simulink model "c1_soft_border"  (R2021b)
settings: Solver=FixedStepDiscrete  StartTime=0.0  StopTime=Inf  FixedStep=sampleTime  RelTol=1e-3  EnableMultiTasking=on
InitFcn:
  | sampleTime = 0.05;
  | nMedianSize=3;
  | % Robot parameters
  | wheelRadius = 0.025;
  | robotRadius = 0.15;
  | 
  | % Lidar parameters
  | sensorOffset = [0,0];
  | scanAngles = linspace(-pi/2,pi/2,9)';
  | maxRange = 5;
  | 
  | %%%%%%
  | ks=-1;
  | 
  | %初始位置
  | x_1_0=0;
  | y_1_0=0;
  | yaw_1_0=0;
  | 
  | x_2_0=0;
  | y_2_0=0.3;
  | yaw_2_0=0;
  | 
  | x_3_0=0;
  | y_3_0=0.6;
  | yaw_3_0=0;
  | 
  | x_4_0=0;
  | y_4_0=0.9;
  | yaw_4_0=0;
  | 
  | 
  | A=0.3;
  | C=1.7;
  | B=(A+C)/2;
  | 
  | wp1=[A,A; B,A;  C,A; C,B;C,C; B,C; A,C;A,B];
  | t=0:0.5:5;
  | Ax=0.8;Ay=0.8;f=2*pi/10;
  | Xd=Ax*sin(2*f*t)+1;
  | Yd=Ay*sin(f*t)+1;
  | WAY_P1=[Xd',Yd'];
  | Ax=0.8;Ay=0.8;f=2*pi/10;
  | Xd=Ax*sin(2*f*t)+1;
  | Yd=-Ay*sin(f*t)+1;
  | WAY_P2=[Xd',Yd'];
  | WAY_P=[WAY_P1(1:end-1,:);WAY_P2(1:end-1,:)];
  | WAY_P=[WAY_P(1:15,:);1,0.5;WAY_P(17:end,:)];
undefined symbols (not defined in the file): Angular, DiscIntNeverNeededParam, Linear
libraries: robotlib x4, dspstat3 x3
settings Model: Creator=The MathWorks, Inc.  LastModifiedBy=FCS
settings SolverCC: AlgebraicLoopSolver=TrustRegion
settings DataIOCC: LimitDataPoints=on  SaveFormat=Array  ReturnWorkspaceOutputs=off
settings OptimizationCC: EnhancedBackFolding=on  PassReuseOutputArgsAs=Individual arguments  ZeroExternalMemoryAtStartup=off  ZeroInternalMemoryAtStartup=off  MaxStackSize=64  OptimizeBlockOrder=speed  DifferentSizesBufferReuse=on  OptimizationCustomize=off  EfficientTunableParamExpr=on
settings DebuggingCC: SolverPrmCheckMsg=warning  ParameterTunabilityLossMsg=error  SFUnexpectedBacktrackingDiag=warning  SFNoUnconditionalDefaultTransitionDiag=warning  SFExecutionAtInitializationDiag=none  SFMachineParentedDataDiag=warning  ArithmeticOperatorsInVariantConditions=warning
settings HardwareCC: ProdBitPerPointer=32  ProdBitPerSizeT=32  ProdBitPerPtrDiffT=32  ProdLargestAtomicFloat=None  ProdIntDivRoundTo=Undefined  ProdEndianess=Unspecified  ProdWordSize=32  ProdHWDeviceType=Generic->Unspecified (assume 32-bit Generic)  TargetHWDeviceType=Generic->Unspecified (assume 32-bit Generic)
settings ModelReferenceCC: PropagateSignalLabelsOutOfModel=off
settings SFSimCC: SimUseLocalCustomCode=off  MATLABDynamicMemAlloc=off  CustomCodeUndefinedFunction=UseInterfaceOnly  SimTargetLang=C++
settings RTWCC: Description=Embedded Coder  SystemTargetFile=ert.tlc  HardwareBoard=Robot Operating System (ROS)  TLCOptions="-aInlineSetEventsForThisBaseRateFcn=TLC_FALSE -aSuppressMultiTaskScheduler=TLC_FALSE  -aRateBasedStepFcn=0"  TemplateMakefile=ert_default_tmf  RTWUseLocalCustomCode=off  Toolchain=Catkin  TargetLang=C++
settings CodeAppCC: ForceParamTrailComments=on  IgnoreCustomStorageClasses=off  OperatorAnnotations=on  SimulinkDataObjDesc=on  SFDataObjDesc=on  InsertBlockDesc=on
settings ERTTargetCC: SupportVariableSizeSignals=on
settings ConfigComp: CovMetricSettings=dw  CovSaveCumulativeToWorkspaceVar=on  CovSaveSingleToWorkspaceVar=on  CovExternalEMLEnable=off  CovSFcnEnable=off

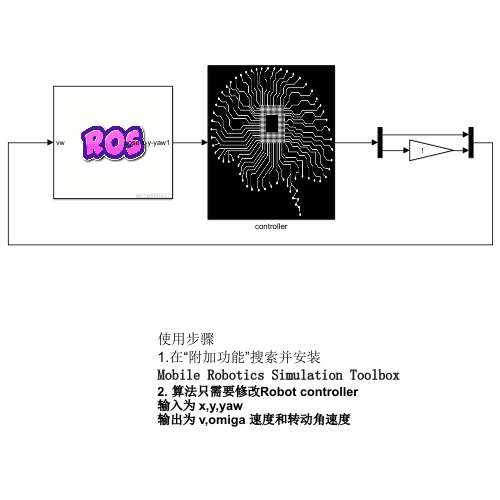
[thumbnail: Simulink's stored preview of the top-level diagram]
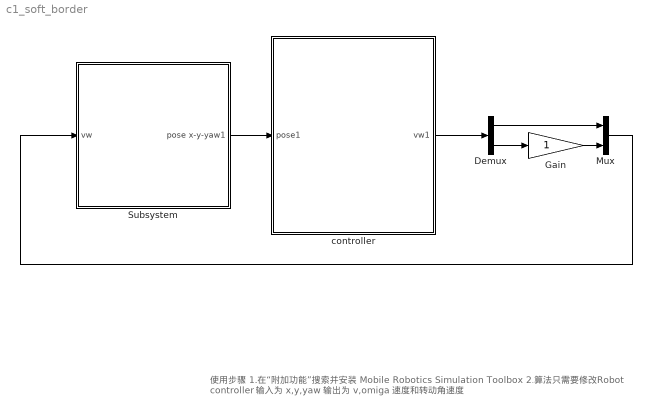
== system c1_soft_border ==
  note: 使用步骤
      | 1.在“附加功能”搜索并安装
      | Mobile Robotics Simulation Toolbox
      | 2. 算法只需要修改Robot controller
      | 输入为 x,y,yaw
      | 输出为 v,omiga 速度和转动角速度
  Demux : Demux  Outputs=2
  Gain : Gain
  Mux : Mux  Inputs=2
  Subsystem : Subsystem
      mask Display: image('$imagefile'); % 使用工具条上的 "编辑图像" 进行更改。
  controller : Subsystem
      mask Display: image('$imagefile'); % 使用工具条上的 "编辑图像" 进行更改。
  wires:
  Mux/1 -> Subsystem/1(vw)
  Gain/1 -> Mux/2
  Subsystem/1(pose x-y-yaw1) -> controller/1(pose1)
  Demux/2 -> Gain/1
  Demux/1 -> Mux/1
  controller/1(vw1) -> Demux/1

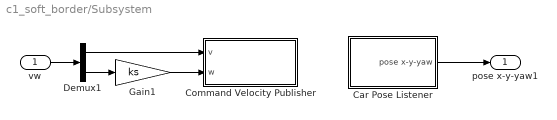
== system c1_soft_border/Subsystem ==
  vw : Inport
  Car Pose Listener : Subsystem
  Command Velocity Publisher : Subsystem
  Demux1 : Demux  Outputs=2
  Gain1 : Gain  Gain=ks
  pose x-y-yaw1 : Outport
  wires:
  vw/1 -> Demux1/1
  Gain1/1 -> Command Velocity Publisher/2(w)
  Demux1/2 -> Gain1/1
  Demux1/1 -> Command Velocity Publisher/1(v)
  Car Pose Listener/1(pose x-y-yaw) -> pose x-y-yaw1/1

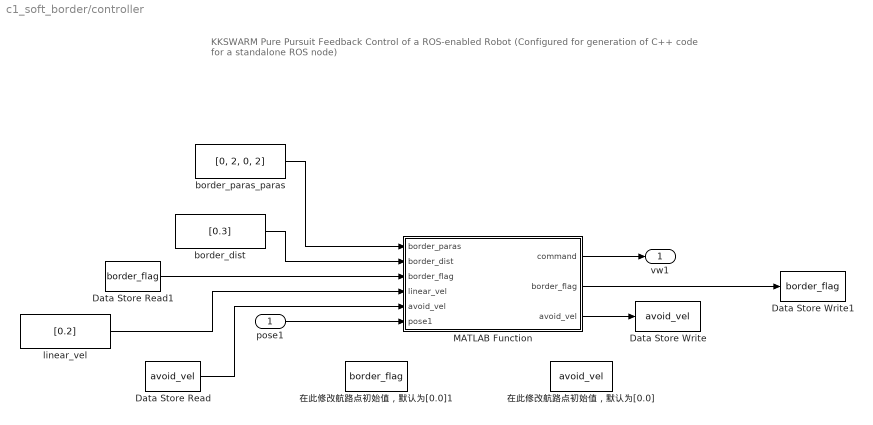
== system c1_soft_border/controller ==
  note: KKSWARM Pure Pursuit Feedback Control of a ROS-enabled Robot
      | (Configured for generation of C++ code for a standalone ROS node)
  pose1 : Inport
  Data Store Read : DataStoreRead  DataStoreName=avoid_vel  IndexOptions=Index vector (dialog)  Indices=1  OutputSizes=1
  Data Store Read1 : DataStoreRead  DataStoreName=border_flag  IndexOptions=Index vector (dialog)  Indices=1  OutputSizes=1
  Data Store Write : DataStoreWrite  DataStoreName=avoid_vel  IndexOptions=Index vector (dialog)  Indices=1  OutputSizes=1
  Data Store Write1 : DataStoreWrite  DataStoreName=border_flag  IndexOptions=Index vector (dialog)  Indices=1  OutputSizes=1
  MATLAB Function : MATLAB Function  TreatAsAtomicUnit=on
  border_dist : Constant  Value=[0.3]  VectorParams1D=off
  border_paras_paras : Constant  Value=[0, 2, 0, 2]  VectorParams1D=off
  linear_vel : Constant  Value=[0.2]  VectorParams1D=off
  在此修改航路点初始值，默认为[0.0] : DataStoreMemory  DataStoreName=avoid_vel  ReadBeforeWriteMsg=warning  WriteAfterWriteMsg=warning  WriteAfterReadMsg=warning  InitialValue=[0.0,0.0]  VectorParams1D=off  ShowAdditionalParam=off
  在此修改航路点初始值，默认为[0.0]1 : DataStoreMemory  DataStoreName=border_flag  ReadBeforeWriteMsg=warning  WriteAfterWriteMsg=warning  WriteAfterReadMsg=warning  InitialValue=[0]  VectorParams1D=off  ShowAdditionalParam=off
  vw1 : Outport
  wires:
  border_dist/1 -> MATLAB Function/2(border_dist)
  Data Store Read1/1 -> MATLAB Function/3("border_flag ")
  Data Store Read/1 -> MATLAB Function/5("avoid_vel ")
  pose1/1 -> MATLAB Function/6(pose1)
  border_paras_paras/1 -> MATLAB Function/1(border_paras)
  linear_vel/1 -> MATLAB Function/4(linear_vel)
  MATLAB Function/2(border_flag) -> Data Store Write1/1
  MATLAB Function/3(avoid_vel) -> Data Store Write/1
  MATLAB Function/1(command) -> vw1/1

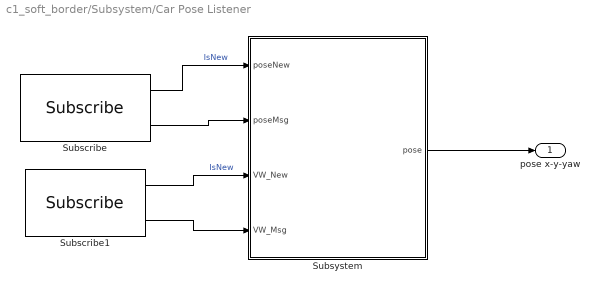
== system c1_soft_border/Subsystem/Car Pose Listener ==
  Subscribe : robotlib/Subscribe  topicSource=Specify your own  topic=/robot_1/pose  messageType=nav_msgs/Odometry  SampleTime=-1  legacyBusStruct=off  messageQueueLength=51
  Subscribe1 : robotlib/Subscribe  topicSource=Specify your own  topic=/robot_1/odometry  messageType=geometry_msgs/Twist  SampleTime=-1  legacyBusStruct=off  messageQueueLength=51
  Subsystem : Subsystem
  pose x-y-yaw : Outport
  wires:
  Subscribe/1 -> Subsystem/1(poseNew)  "IsNew"
  Subscribe/2 -> Subsystem/2(poseMsg)
  Subscribe1/1 -> Subsystem/3(VW_New)  "IsNew"
  Subscribe1/2 -> Subsystem/4(VW_Msg)
  Subsystem/1(pose) -> pose x-y-yaw/1

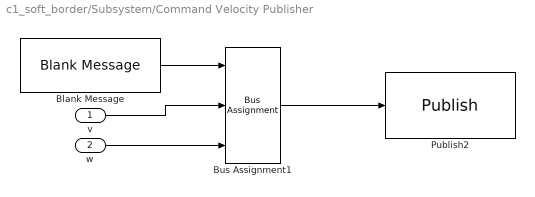
== system c1_soft_border/Subsystem/Command Velocity Publisher ==
  v : Inport
  w : Inport  Port=2
  Blank Message : robotlib/Blank Message  messageClass=Message  entityType=geometry_msgs/Twist  messageType=geometry_msgs/Twist  SampleTime=inf  legacyBusStruct=off
  Bus Assignment1 : BusAssignment  DialogController=Simulink.DDGSource_BusAssignment  AssignedSignals=Linear.X,Angular.Z
  Publish2 : robotlib/Publish  topicSource=Specify your own  topic=/robot_1/cmd_vel  messageType=geometry_msgs/Twist  legacyBusStruct=off  messageQueueLength=105
  wires:
  Bus Assignment1/1 -> Publish2/1
  Blank Message/1 -> Bus Assignment1/1
  v/1 -> Bus Assignment1/2
  w/1 -> Bus Assignment1/3

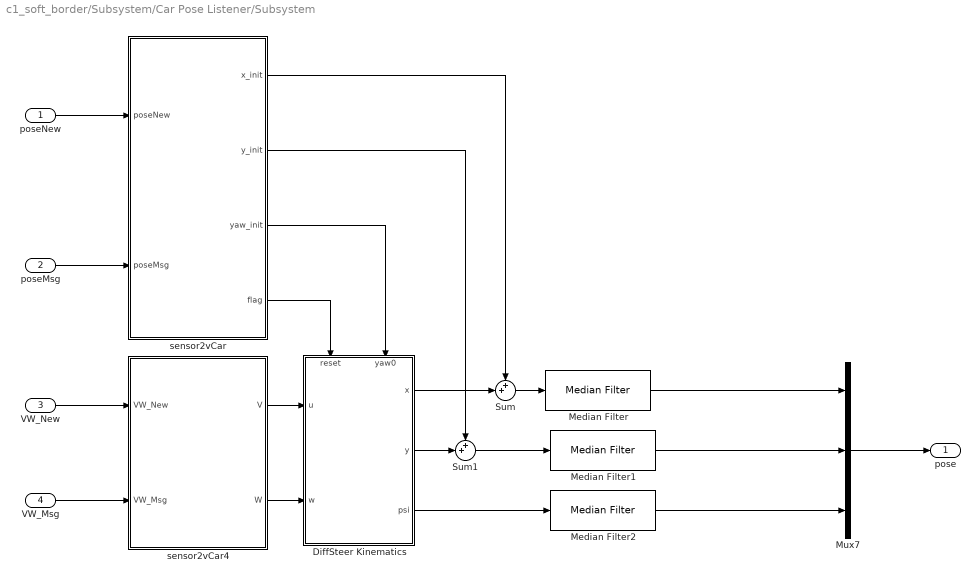
== system c1_soft_border/Subsystem/Car Pose Listener/Subsystem ==
  poseNew : Inport
  poseMsg : Inport  Port=2
  VW_New : Inport  Port=3
  VW_Msg : Inport  Port=4
  DiffSteer Kinematics : Subsystem
      settings: PortSchema="{\"entries\":[{\"content\":{\"sides\":[{\"content\":{\"connectorIds\":[\"In1\",\"In2\"]},\"type\":\"ConnectorPlacement.EquallySpacedRectSide\",\"uuid\":\"0032ed68-1de4-4b1c-b237-9372fedc8a7a\"},{\"content\":{\"connectorIds\":[\"Out1\",\"Out2\",\"Out3\"],\"side\":\"RIGHT\"},\"type\":\"ConnectorPlacement.EquallySpacedRectSide\",\"uuid\":\"d0c861bd-7497-47fe-b183-36da470ee2c6\"},{\"content\":{\"connectorIds\":[\"In3\",\"In4\"],\"side\":\"TOP\"},\"type\":\"ConnectorPlacement.EquallySpacedRectSide\",\"uuid\":\"5b685229-150b-4cb5-b33d-c61d28c4627e\"}]},\"type\":\"ConnectorPlacement.EquallySpacedConnector\",\"uuid\":\"4513c50b-5820-40cb-bb28-cc7c1b1322fe\"}],\"packageUris\":[\"http://schema.mathworks.com/mf0/Connector/R2020b\"],\"version\":\"1.0\"}"
  Median Filter : dspstat3/Median Filter  WindowLength=nMedianSize  SimulateUsing=Interpreted execution
      settings: SourceProductBaseCode=DS
  Median Filter1 : dspstat3/Median Filter  WindowLength=nMedianSize  SimulateUsing=Interpreted execution
      settings: SourceProductBaseCode=DS
  Median Filter2 : dspstat3/Median Filter  WindowLength=nMedianSize  SimulateUsing=Interpreted execution
      settings: SourceProductBaseCode=DS
  Mux7 : Mux  Inputs=3
  Sum : Sum  Inputs=++|
  Sum1 : Sum  Inputs=++|
  sensor2vCar : MATLAB Function  TreatAsAtomicUnit=on
  sensor2vCar4 : MATLAB Function  TreatAsAtomicUnit=on
  pose : Outport
  wires:
  Median Filter2/1 -> Mux7/3
  Median Filter1/1 -> Mux7/2
  Median Filter/1 -> Mux7/1
  sensor2vCar/4(flag) -> DiffSteer Kinematics/3(reset)
  DiffSteer Kinematics/2(y) -> Sum1/2
  sensor2vCar/3(yaw_init) -> DiffSteer Kinematics/4(yaw0)
  sensor2vCar/2(y_init) -> Sum1/1
  sensor2vCar/1(x_init) -> Sum/1
  DiffSteer Kinematics/1(x) -> Sum/2
  VW_New/1 -> sensor2vCar4/1(VW_New)
  Mux7/1 -> pose/1
  Sum/1 -> Median Filter/1
  DiffSteer Kinematics/3(psi) -> Median Filter2/1
  sensor2vCar4/1(V) -> DiffSteer Kinematics/1(u)
  Sum1/1 -> Median Filter1/1
  sensor2vCar4/2(W) -> DiffSteer Kinematics/2(w)
  poseNew/1 -> sensor2vCar/1(poseNew)
  poseMsg/1 -> sensor2vCar/2(poseMsg)
  VW_Msg/1 -> sensor2vCar4/2(VW_Msg)

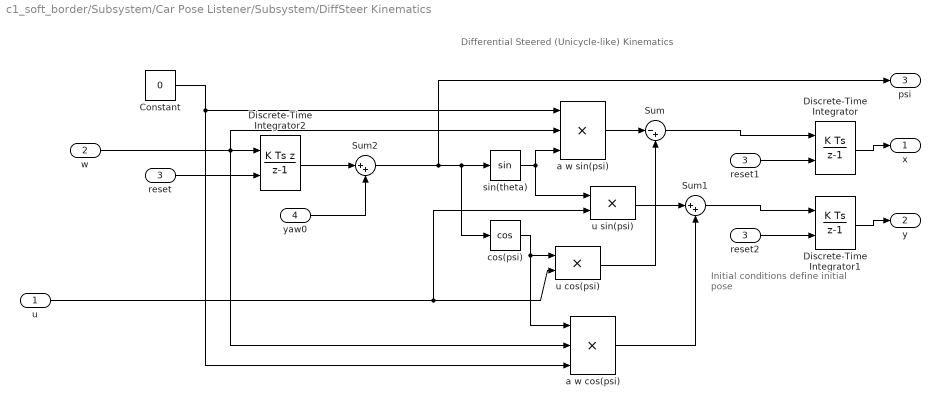
== system c1_soft_border/Subsystem/Car Pose Listener/Subsystem/DiffSteer Kinematics ==
  note: Initial conditions define
      | initial pose
  note: Differential Steered (Unicycle-like) Kinematics
  u : Inport
  w : Inport  Port=2
  reset : Inport  Port=3
  yaw0 : Inport  Port=4
  Constant : Constant  Value=0
  Discrete-Time Integrator : DiscreteIntegrator  ExternalReset=falling  SampleTime=-1  ICPrevOutput=DiscIntNeverNeededParam  ICPrevScaledInput=DiscIntNeverNeededParam
  Discrete-Time Integrator1 : DiscreteIntegrator  ExternalReset=falling  SampleTime=-1  ICPrevOutput=DiscIntNeverNeededParam  ICPrevScaledInput=DiscIntNeverNeededParam
  Discrete-Time Integrator2 : DiscreteIntegrator  IntegratorMethod=Integration: Backward Euler  ExternalReset=falling  SampleTime=-1  ICPrevOutput=DiscIntNeverNeededParam  ICPrevScaledInput=DiscIntNeverNeededParam
  Sum : Sum  Inputs=|-+  SaturateOnIntegerOverflow=on
  Sum1 : Sum  Inputs=|++  SaturateOnIntegerOverflow=on
  Sum2 : Sum  Inputs=|++
  a w cos(psi) : Product  Inputs=3  SaturateOnIntegerOverflow=on  OutDataTypeStr=Inherit: Same as first input
  a w sin(psi) : Product  Inputs=3  SaturateOnIntegerOverflow=on  OutDataTypeStr=Inherit: Same as first input
  cos(psi) : Trigonometry  Operator=cos
  reset1 : InportShadow  Port=3
  reset2 : InportShadow  Port=3
  sin(theta) : Trigonometry
  u cos(psi) : Product  SaturateOnIntegerOverflow=on  OutDataTypeStr=Inherit: Same as first input
  u sin(psi) : Product  SaturateOnIntegerOverflow=on  OutDataTypeStr=Inherit: Same as first input
  x : Outport
  y : Outport  Port=2
  psi : Outport  Port=3
  wires:
  yaw0/1 -> Sum2/2
  reset2/1 -> Discrete-Time Integrator1/2
  reset1/1 -> Discrete-Time Integrator/2
  reset/1 -> Discrete-Time Integrator2/2
  u sin(psi)/1 -> Sum1/1
  cos(psi)/1 -> u cos(psi)/1, a w cos(psi)/1
  w/1 -> a w cos(psi)/2, a w sin(psi)/2, Discrete-Time Integrator2/1
  Constant/1 -> a w sin(psi)/1, a w cos(psi)/3
  Discrete-Time Integrator/1 -> x/1
  Sum/1 -> Discrete-Time Integrator/1
  sin(theta)/1 -> a w sin(psi)/3, u sin(psi)/1
  a w cos(psi)/1 -> Sum1/2
  Sum2/1 -> psi/1, sin(theta)/1, cos(psi)/1
  u cos(psi)/1 -> Sum/2
  u/1 -> u sin(psi)/2, u cos(psi)/2
  a w sin(psi)/1 -> Sum/1
  Sum1/1 -> Discrete-Time Integrator1/1
  Discrete-Time Integrator1/1 -> y/1
  Discrete-Time Integrator2/1 -> Sum2/1

== matlab function c1_soft_border/controller/MATLAB Function ==
  settings: updateMethod=DISCRETE
  data: border_paras input; border_dist input; border_flag input; linear_vel input; avoid_vel input; pose1 input; command output; border_flag output; avoid_vel output
function [command,border_flag, avoid_vel] = car1(border_paras, border_dist, border_flag, linear_vel, avoid_vel, pose1)

%%%%% input
x=pose1(1);
y=pose1(2);
yaw=pose1(3);

% 将航向角转换成0,2pi
yaw = yaw - floor(yaw/(2*3.1415926))*2*3.1415926 + 2*3.1415926;

if yaw >= 2*3.1415926
    yaw = yaw - 2*3.1415926;
end

current_flag = is_in_border(border_paras, border_dist, x, y);

if current_flag == 0
    w = -1 + 2 * rand();
    command = [linear_vel, 0.0];
    avoid_vel = [0.0, 0.0];

else
    [v, w, avoid_vel] = border_avoid(border_paras, border_dist, linear_vel, border_flag, current_flag, avoid_vel, x, y, yaw)
    command = [v, w];
end
border_flag = current_flag;
end

function flag = is_in_border(border_paras, border_dist, x, y)
    flag =0;

    x_low = border_paras(1) + border_dist;
    x_high = border_paras(2) - border_dist;

    y_low = border_paras(3) + border_dist;
    y_high = border_paras(4) - border_dist;

    if x >= x_high
        flag = 1;
    end

    if x <= x_low
        flag = 2;
    end

    if y >= y_high 
        flag = 3;
    end


    if y <= y_low
        flag = 4;
    end

end 

function [v, w, avoid_vel] = border_avoid(border_paras, border_dist, linear_vel, border_flag, current_flag, avoid_vel, x, y, yaw)
    x_low = border_paras(1) + border_dist;
    x_high = border_paras(2) - border_dist;

    y_low = border_paras(3) + border_dist;
    y_high = border_paras(4) - border_dist;

    if border_flag>0 && current_flag>0 && border_flag~=current_flag
        avoid_vel = [0.0, 0.0];
    end

    if avoid_vel(1)==0.0 && avoid_vel(2)==0.0
        vx = linear_vel * cos(yaw);
        vy = linear_vel * sin(yaw);
    
        % 右边界
        if x >= x_high
            if vx>=0
                vx = -vx;
            end
        end
    
        % 左边界
        if x <= x_low
            if vx < 0
                vx = -vx;
            end
        end
    
        % 上边界
        if y >= y_high
            if vy >=0 
                vy = -vy;
            end
        end
    
        % 下边界
        if y <= y_low
            if vy < 0
                vy = -vy;
            end
        end

        avoid_vel = [vx, vy];

    end
    
    % 计算期望航向角(度)
    new_yaw = atan2(avoid_vel(2), avoid_vel(1))*180.0/3.1415926;
    
    if new_yaw < 0
        new_yaw = 360.0 + new_yaw;
    end

    delta_theta = new_yaw - yaw*180.0/3.1415926;

    if delta_theta > 180.0
        delta_theta =  delta_theta - 360.0;
    end

    if delta_theta < -180.0
        delta_theta = delta_theta + 360.0;
    end

    kk = 1.0;

    max_angular_speed = 2.0;

    angular_speed = kk * delta_theta * 3.1415926 / 180.0;

    if angular_speed > max_angular_speed
        angular_speed = max_angular_speed;
    end

    if angular_speed < -max_angular_speed
        angular_speed = -max_angular_speed;
    end

    v = linear_vel;
    w = angular_speed;

end

== matlab function c1_soft_border/Subsystem/Car Pose Listener/Subsystem/sensor2vCar ==
  data: x_init output; y_init output; yaw_init output; flag output; poseNew input; poseMsg input
function [x_init,y_init,yaw_init,flag] = sensor2vCar(poseNew, poseMsg)
persistent x0 y0 yaw0 yaw1 x0_init y0_init yaw0_init fStart
if isempty(x0)
    x0=-10; y0=-10; yaw0=0; yaw1=0;   
    x0_init=-10;y0_init=-10;yaw0_init=0;
    fStart=0;
end
if poseNew
    if x0==poseMsg.Pose.Pose.Position.X&&y0==poseMsg.Pose.Pose.Position.Y
        flag=1;
    else
        x0=poseMsg.Pose.Pose.Position.X;
        y0=poseMsg.Pose.Pose.Position.Y;   
        %yaw2=atan2(2*(poseMsg.Pose.Pose.Orientation.Z*poseMsg.Pose.Pose.Orientation.W),1-2*(poseMsg.Pose.Pose.Orientation.Z^2)); 
        eul=quat2eul([poseMsg.Pose.Pose.Orientation.W,poseMsg.Pose.Pose.Orientation.X,poseMsg.Pose.Pose.Orientation.Y,poseMsg.Pose.Pose.Orientation.Z]);
        yaw2=eul(1);
        %对前后角度差使用积分，恢复yaw的连续性
        yaw0=yaw0+angdiff(yaw1,yaw2);
        yaw1=yaw2;
        flag=0;        
        x0_init=x0;
        y0_init=y0;
        yaw0_init=yaw0;
        fStart=1;
    end 
else
    if fStart
        flag=1;
    else
        flag=0;
    end
end

x_init=x0_init;y_init=y0_init;yaw_init=yaw0_init;

== matlab function c1_soft_border/Subsystem/Car Pose Listener/Subsystem/sensor2vCar4 ==
  data: V output; W output; VW_New input; VW_Msg input
function [V,W] = sensor2vCar(VW_New, VW_Msg)
persistent v0 w0
if isempty(v0)
    v0=0; 
    w0=0;    
end
if VW_New
    v0=VW_Msg.Linear.X;
    w0=VW_Msg.Angular.Z;
end

V=v0;
W=-w0;
